simulink model "subsystems_enable_triggered"  (R2022b)
settings: Solver=FixedStepAuto  StartTime=0.0  StopTime=10.0  FixedStep=1e-3  RelTol=1e-3
settings Model: Creator=yasso  LastModifiedBy=yasso
settings DebuggingCC: UnconnectedInputMsg=warning  UnconnectedOutputMsg=warning  UnconnectedLineMsg=warning
settings ModelReferenceCC: EnableRefExpFcnMdlSchedulingChecks=on
settings RTWCC: DLArmComputeVersion=19.05

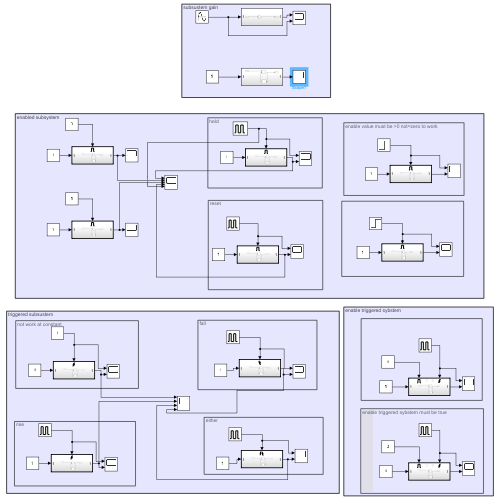
[thumbnail: Simulink's stored preview of the top-level diagram]
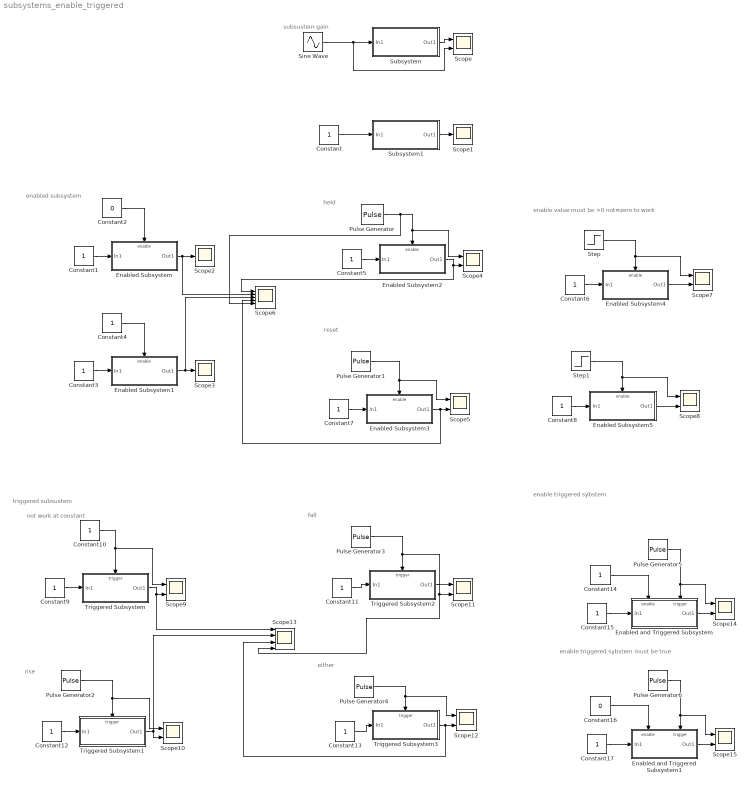
== system subsystems_enable_triggered ==
  note: enable triggered sybstem
  note: enable triggered sybstem must be true
  note: triggered subsustem
  note: fall
  note: rise
  note: not work at constant
  note: enable value must be >0 not=zero to work
  note: held
  note: reset
  note: enabled subsystem
  note: subsustem gain
  note: either
  Constant{,1,3..15,17} (16 alike) : Constant
  Constant16 : Constant  Value=0
  Constant2 : Constant  Value=0
  Enabled Subsystem : Subsystem  TreatAsAtomicUnit=on
  Enabled Subsystem1 : Subsystem  TreatAsAtomicUnit=on
  Enabled Subsystem2 : Subsystem  TreatAsAtomicUnit=on
  Enabled Subsystem3 : Subsystem  TreatAsAtomicUnit=on
  Enabled Subsystem4 : Subsystem  TreatAsAtomicUnit=on
  Enabled Subsystem5 : Subsystem  TreatAsAtomicUnit=on
  Enabled and Triggered Subsystem : Subsystem  TreatAsAtomicUnit=on
  Enabled and Triggered Subsystem1 : Subsystem  TreatAsAtomicUnit=on
  Pulse Generator : DiscretePulseGenerator  PulseType=Time based  PulseWidth=50
  Pulse Generator1 : DiscretePulseGenerator  PulseType=Time based  PulseWidth=50
  Pulse Generator{2..6} (5 alike) : DiscretePulseGenerator  PulseType=Time based  PulseWidth=5
  Scope{,4..5,7..12,14..15} (11 alike) : Scope  NumInputPorts=2
  Scope1 : Scope
  Scope13 : Scope  NumInputPorts=4
  Scope2 : Scope
  Scope3 : Scope
  Scope6 : Scope  NumInputPorts=5
  Sine Wave : Sin  SampleTime=0
  Step : Step  Before=-1  After=0  SampleTime=0
  Step1 : Step  Before=-1  SampleTime=0
  Subsystem : Subsystem
  Subsystem1 : Subsystem
  Triggered Subsystem : Subsystem  TreatAsAtomicUnit=on
  Triggered Subsystem1 : Subsystem  TreatAsAtomicUnit=on
  Triggered Subsystem2 : Subsystem  TreatAsAtomicUnit=on
  Triggered Subsystem3 : Subsystem  TreatAsAtomicUnit=on
  wires:
  Sine Wave/1 -> Scope/2, Subsystem/1(In1)
  Subsystem/1(Out1) -> Scope/1
  Constant/1 -> Subsystem1/1(In1)
  Subsystem1/1(Out1) -> Scope1/1
  Constant1/1 -> Enabled Subsystem/1(In1)
  Enabled Subsystem/1(Out1) -> Scope6/2, Scope2/1
  Constant2/1 -> Enabled Subsystem/Enable
  Enabled Subsystem1/1(Out1) -> Scope6/3, Scope3/1
  Constant3/1 -> Enabled Subsystem1/1(In1)
  Constant4/1 -> Enabled Subsystem1/Enable
  Enabled Subsystem2/1(Out1) -> Scope6/1, Scope4/2
  Pulse Generator1/1 -> Scope5/1, Enabled Subsystem3/Enable
  Constant5/1 -> Enabled Subsystem2/1(In1)
  Pulse Generator/1 -> Scope6/5, Scope4/1, Enabled Subsystem2/Enable
  Enabled Subsystem3/1(Out1) -> Scope6/4, Scope5/2
  Constant7/1 -> Enabled Subsystem3/1(In1)
  Step/1 -> Scope7/1, Enabled Subsystem4/Enable
  Constant6/1 -> Enabled Subsystem4/1(In1)
  Enabled Subsystem4/1(Out1) -> Scope7/2
  Step1/1 -> Scope8/1, Enabled Subsystem5/Enable
  Enabled Subsystem5/1(Out1) -> Scope8/2
  Constant8/1 -> Enabled Subsystem5/1(In1)
  Constant10/1 -> Scope9/1, Triggered Subsystem/Trigger
  Constant9/1 -> Triggered Subsystem/1(In1)
  Triggered Subsystem/1(Out1) -> Scope13/1, Scope9/2
  Triggered Subsystem1/1(Out1) -> Scope10/2, Scope13/2
  Constant12/1 -> Triggered Subsystem1/1(In1)
  Pulse Generator2/1 -> Scope10/1, Triggered Subsystem1/Trigger
  Pulse Generator3/1 -> Triggered Subsystem2/Trigger, Scope11/1
  Constant11/1 -> Triggered Subsystem2/1(In1)
  Triggered Subsystem2/1(Out1) -> Scope11/2, Scope13/4
  Constant13/1 -> Triggered Subsystem3/1(In1)
  Triggered Subsystem3/1(Out1) -> Scope13/3, Scope12/2
  Pulse Generator4/1 -> Triggered Subsystem3/Trigger, Scope12/1
  Constant14/1 -> Enabled and Triggered Subsystem/Enable
  Pulse Generator5/1 -> Scope14/1, Enabled and Triggered Subsystem/Trigger
  Constant15/1 -> Enabled and Triggered Subsystem/1(In1)
  Enabled and Triggered Subsystem/1(Out1) -> Scope14/2
  Enabled and Triggered Subsystem1/1(Out1) -> Scope15/2
  Constant17/1 -> Enabled and Triggered Subsystem1/1(In1)
  Pulse Generator6/1 -> Enabled and Triggered Subsystem1/Trigger, Scope15/1
  Constant16/1 -> Enabled and Triggered Subsystem1/Enable

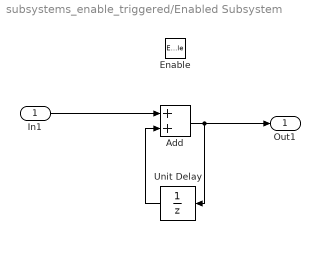
== system subsystems_enable_triggered/Enabled Subsystem ==
  In1 : Inport
  Enable : EnablePort
  Add : Sum
  Unit Delay : UnitDelay  SampleTime=-1  HasFrameUpgradeWarning=on
  Out1 : Outport
  wires:
  Add/1 -> Unit Delay/1, Out1/1
  Unit Delay/1 -> Add/2
  In1/1 -> Add/1

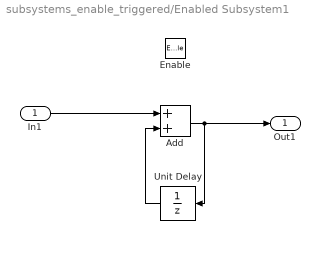
== system subsystems_enable_triggered/Enabled Subsystem1 ==
  In1 : Inport
  Enable : EnablePort
  Add : Sum
  Unit Delay : UnitDelay  SampleTime=-1  HasFrameUpgradeWarning=on
  Out1 : Outport
  wires:
  Add/1 -> Unit Delay/1, Out1/1
  Unit Delay/1 -> Add/2
  In1/1 -> Add/1

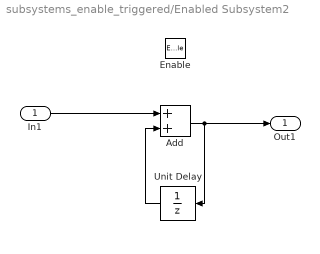
== system subsystems_enable_triggered/Enabled Subsystem2 ==
  In1 : Inport
  Enable : EnablePort
  Add : Sum
  Unit Delay : UnitDelay  SampleTime=-1  HasFrameUpgradeWarning=on
  Out1 : Outport
  wires:
  Add/1 -> Unit Delay/1, Out1/1
  Unit Delay/1 -> Add/2
  In1/1 -> Add/1

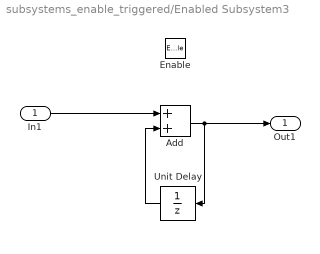
== system subsystems_enable_triggered/Enabled Subsystem3 ==
  In1 : Inport
  Enable : EnablePort  StatesWhenEnabling=reset
  Add : Sum
  Unit Delay : UnitDelay  SampleTime=-1  HasFrameUpgradeWarning=on
  Out1 : Outport
  wires:
  Add/1 -> Unit Delay/1, Out1/1
  Unit Delay/1 -> Add/2
  In1/1 -> Add/1

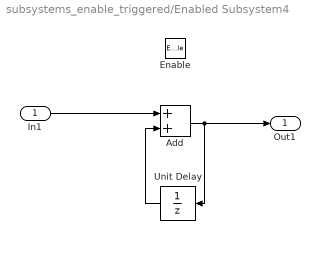
== system subsystems_enable_triggered/Enabled Subsystem4 ==
  In1 : Inport
  Enable : EnablePort
  Add : Sum
  Unit Delay : UnitDelay  SampleTime=-1  HasFrameUpgradeWarning=on
  Out1 : Outport
  wires:
  Add/1 -> Unit Delay/1, Out1/1
  Unit Delay/1 -> Add/2
  In1/1 -> Add/1

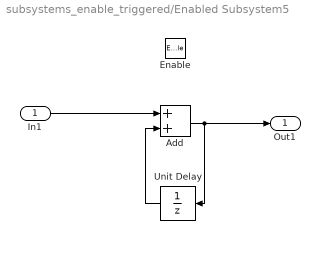
== system subsystems_enable_triggered/Enabled Subsystem5 ==
  In1 : Inport
  Enable : EnablePort
  Add : Sum
  Unit Delay : UnitDelay  SampleTime=-1  HasFrameUpgradeWarning=on
  Out1 : Outport
  wires:
  Add/1 -> Unit Delay/1, Out1/1
  Unit Delay/1 -> Add/2
  In1/1 -> Add/1

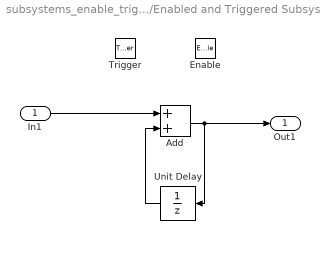
== system subsystems_enable_triggered/Enabled and Triggered Subsystem ==
  In1 : Inport
  Enable : EnablePort
  Trigger : TriggerPort  VariantControl=(inherit)
  Add : Sum
  Unit Delay : UnitDelay  SampleTime=-1  HasFrameUpgradeWarning=on
  Out1 : Outport
  wires:
  Add/1 -> Out1/1, Unit Delay/1
  In1/1 -> Add/1
  Unit Delay/1 -> Add/2

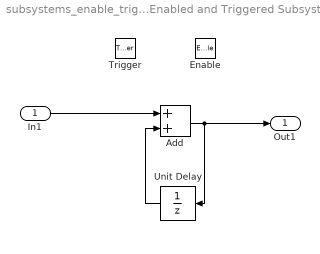
== system subsystems_enable_triggered/Enabled and Triggered Subsystem1 ==
  In1 : Inport
  Enable : EnablePort
  Trigger : TriggerPort  VariantControl=(inherit)
  Add : Sum
  Unit Delay : UnitDelay  SampleTime=-1  HasFrameUpgradeWarning=on
  Out1 : Outport
  wires:
  Unit Delay/1 -> Add/2
  In1/1 -> Add/1
  Add/1 -> Unit Delay/1, Out1/1

== system subsystems_enable_triggered/Subsystem ==
  In1 : Inport
  Gain : Gain  Gain=3
  Out1 : Outport
  wires:
  In1/1 -> Gain/1
  Gain/1 -> Out1/1

== system subsystems_enable_triggered/Subsystem1 ==
  In1 : Inport
  Add : Sum
  Unit Delay : UnitDelay  SampleTime=-1  HasFrameUpgradeWarning=on
  Out1 : Outport
  wires:
  In1/1 -> Add/1
  Add/1 -> Unit Delay/1, Out1/1
  Unit Delay/1 -> Add/2

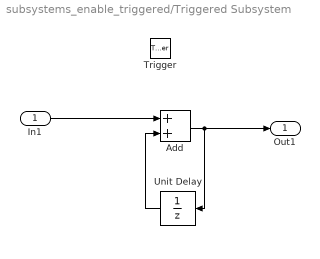
== system subsystems_enable_triggered/Triggered Subsystem ==
  In1 : Inport
  Trigger : TriggerPort  VariantControl=(inherit)
  Add : Sum
  Unit Delay : UnitDelay  SampleTime=-1  HasFrameUpgradeWarning=on
  Out1 : Outport
  wires:
  Unit Delay/1 -> Add/2
  In1/1 -> Add/1
  Add/1 -> Unit Delay/1, Out1/1

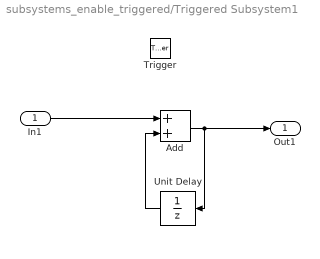
== system subsystems_enable_triggered/Triggered Subsystem1 ==
  In1 : Inport
  Trigger : TriggerPort  VariantControl=(inherit)
  Add : Sum
  Unit Delay : UnitDelay  SampleTime=-1  HasFrameUpgradeWarning=on
  Out1 : Outport
  wires:
  Unit Delay/1 -> Add/2
  In1/1 -> Add/1
  Add/1 -> Unit Delay/1, Out1/1

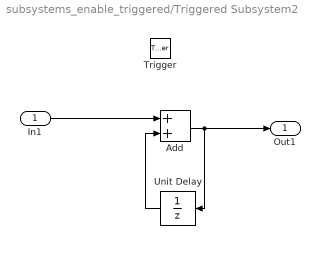
== system subsystems_enable_triggered/Triggered Subsystem2 ==
  In1 : Inport
  Trigger : TriggerPort  TriggerType=falling  VariantControl=(inherit)
  Add : Sum
  Unit Delay : UnitDelay  SampleTime=-1  HasFrameUpgradeWarning=on
  Out1 : Outport
  wires:
  Add/1 -> Out1/1, Unit Delay/1
  In1/1 -> Add/1
  Unit Delay/1 -> Add/2

== system subsystems_enable_triggered/Triggered Subsystem3 ==
  In1 : Inport
  Trigger : TriggerPort  TriggerType=either  VariantControl=(inherit)
  Add : Sum
  Unit Delay : UnitDelay  SampleTime=-1  HasFrameUpgradeWarning=on
  Out1 : Outport
  wires:
  Add/1 -> Out1/1, Unit Delay/1
  In1/1 -> Add/1
  Unit Delay/1 -> Add/2
